simulink model "Complementary_filter_Sim"  (R2024b)
settings: Solver=ode4  StartTime=0.0  StopTime=10.0  FixedStep=0.01  RelTol=1e-3
undefined symbols (not defined in the file): C1, C2, C3, g0, H_initial, Omega_S
settings Model: Creator=JUN  LastModifiedBy=JUN

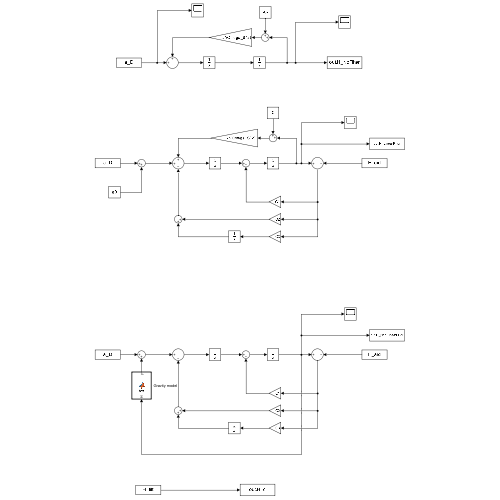
[thumbnail: Simulink's stored preview of the top-level diagram]
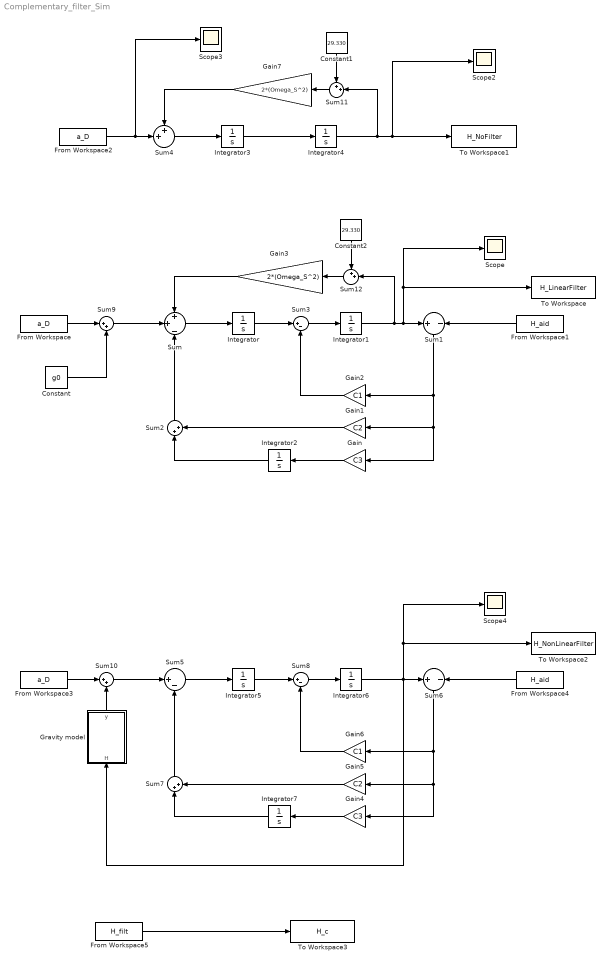
== system Complementary_filter_Sim ==
  Constant : Constant  Value=g0
  Constant1 : Constant  Value=29.330
  Constant2 : Constant  Value=29.330
  From Workspace : FromWorkspace  VariableName=a_D
  From Workspace1 : FromWorkspace  VariableName=H_aid
  From Workspace2 : FromWorkspace  VariableName=a_D
  From Workspace3 : FromWorkspace  VariableName=a_D
  From Workspace4 : FromWorkspace  VariableName=H_aid
  From Workspace5 : FromWorkspace  VariableName=H_filt
  Gain : Gain  Gain=C3
  Gain1 : Gain  Gain=C2
  Gain2 : Gain  Gain=C1
  Gain3 : Gain  Gain=2*(Omega_S^2)
  Gain4 : Gain  Gain=C3
  Gain5 : Gain  Gain=C2
  Gain6 : Gain  Gain=C1
  Gain7 : Gain  Gain=2*(Omega_S^2)
  Gravity model : MATLAB Function  TreatAsAtomicUnit=on
  Integrator{,2..3,5,7} (5 alike) : Integrator
  Integrator1 : Integrator  InitialCondition=H_initial
  Integrator4 : Integrator  InitialCondition=H_initial
  Integrator6 : Integrator  InitialCondition=H_initial
  Scope{,2..4} (4 alike) : Scope
  Sum : Sum  Inputs=+|+|-
  Sum1 : Sum  Inputs=+-
  Sum{2,7,9..10} (4 alike) : Sum  Inputs=|++
  Sum11 : Sum  Inputs=++|
  Sum12 : Sum  Inputs=++|
  Sum3 : Sum  Inputs=|+-
  Sum4 : Sum  Inputs=++|
  Sum5 : Sum  Inputs=|+-
  Sum6 : Sum  Inputs=+-
  Sum8 : Sum  Inputs=|+-
  To Workspace : ToWorkspace  VariableName=H_LinearFilter  SampleTime=-1
  To Workspace1 : ToWorkspace  VariableName=H_NoFilter  SampleTime=-1
  To Workspace2 : ToWorkspace  VariableName=H_NonLinearFilter  SampleTime=-1
  To Workspace3 : ToWorkspace  VariableName=H_c  SampleTime=-1
  wires:
  Sum/1 -> Integrator/1
  Integrator1/1 -> Sum12/2, Scope/1, To Workspace/1, Sum1/1
  Sum1/1 -> Gain/1, Gain1/1, Gain2/1
  Integrator/1 -> Sum3/1
  Sum3/1 -> Integrator1/1
  Gain1/1 -> Sum2/2
  Gain/1 -> Integrator2/1
  Integrator2/1 -> Sum2/1
  Gain3/1 -> Sum/1
  Integrator4/1 -> Sum11/2, Scope2/1, To Workspace1/1
  Integrator3/1 -> Integrator4/1
  From Workspace2/1 -> Scope3/1, Sum4/2
  Gain7/1 -> Sum4/1
  Sum4/1 -> Integrator3/1
  From Workspace1/1 -> Sum1/2
  Sum2/1 -> Sum/3
  Gain2/1 -> Sum3/2
  Gain6/1 -> Sum8/2
  From Workspace4/1 -> Sum6/2
  Integrator6/1 -> Gravity model/1(H), Scope4/1, To Workspace2/1, Sum6/1
  Sum8/1 -> Integrator6/1
  Gain5/1 -> Sum7/2
  Sum6/1 -> Gain4/1, Gain5/1, Gain6/1
  Gain4/1 -> Integrator7/1
  Integrator7/1 -> Sum7/1
  Integrator5/1 -> Sum8/1
  Sum5/1 -> Integrator5/1
  From Workspace/1 -> Sum9/1
  Constant/1 -> Sum9/2
  Sum9/1 -> Sum/2
  From Workspace3/1 -> Sum10/1
  Gravity model/1(y) -> Sum10/2
  Sum7/1 -> Sum5/2
  Sum10/1 -> Sum5/1
  From Workspace5/1 -> To Workspace3/1
  Sum11/1 -> Gain7/1
  Constant1/1 -> Sum11/1
  Constant2/1 -> Sum12/1
  Sum12/1 -> Gain3/1

== matlab function Complementary_filter_Sim/Gravity model ==
  data: H input; y output
function y = fcn(H)

h = H + 29.330;

y = -9.7983/((1 + (h/6378137))^2);
